simulink model "Manual_Simu_2022a"  (R2022a)
settings: Solver=VariableStepAuto  StartTime=0.0  StopTime=3  RelTol=1e-3
values from neighbouring files (symbols this model uses):
  c = 0.9    [Mechatronics_System.m]
  g = 9.81    [Mechatronics_System.m]
  I_p = (1/3)*m_p*l^2    (= 2.35225)    [Mechatronics_System.m]
  l = 0.97    [Mechatronics_System.m]
  m_p = 7.5    [Mechatronics_System.m]
  m_w = 30.5    [Mechatronics_System.m]
libraries: simulink_extras x2, simulink x1
settings Model: Creator=sango  LastModifiedBy=sango
settings DebuggingCC: ArtificialAlgebraicLoopMsg=none
settings ModelReferenceCC: EnableRefExpFcnMdlSchedulingChecks=off
settings RTWCC: Description=Generic Real-Time Target

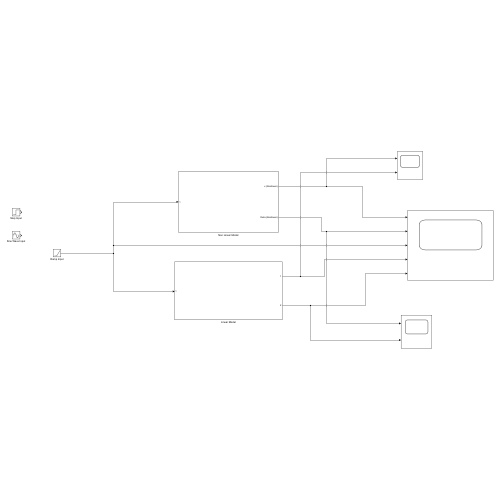
[thumbnail: Simulink's stored preview of the top-level diagram]
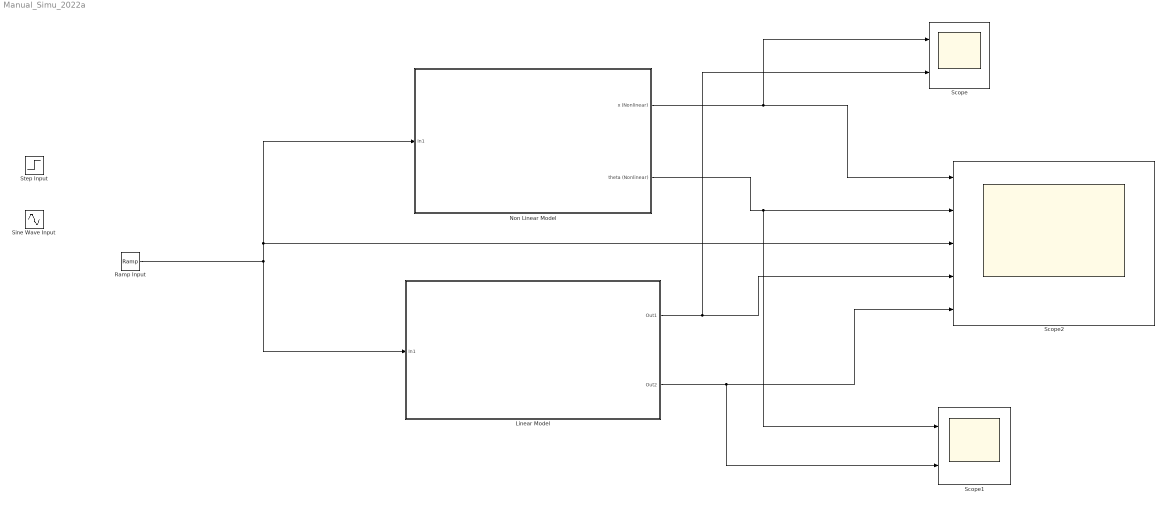
== system Manual_Simu_2022a ==
  Linear Model : Subsystem
  Non Linear Model : Subsystem
  Ramp Input : simulink/Sources/Ramp  slope=2  start=0  InitialOutput=0
  Scope : Scope  NumInputPorts=2
  Scope1 : Scope  NumInputPorts=2
  Scope2 : Scope  NumInputPorts=5
  Sine Wave Input : Sin  SampleTime=0
  Step Input : Step  SampleTime=0
  wires:
  Non Linear Model/1(x (Nonlinear)) -> Scope/1, Scope2/1
  Non Linear Model/2(theta (Nonlinear)) -> Scope1/1, Scope2/2
  Ramp Input/1 -> Linear Model/1(In1), Scope2/3, Non Linear Model/1(In1)
  Linear Model/1(Out1) -> Scope/2, Scope2/4
  Linear Model/2(Out2) -> Scope1/2, Scope2/5

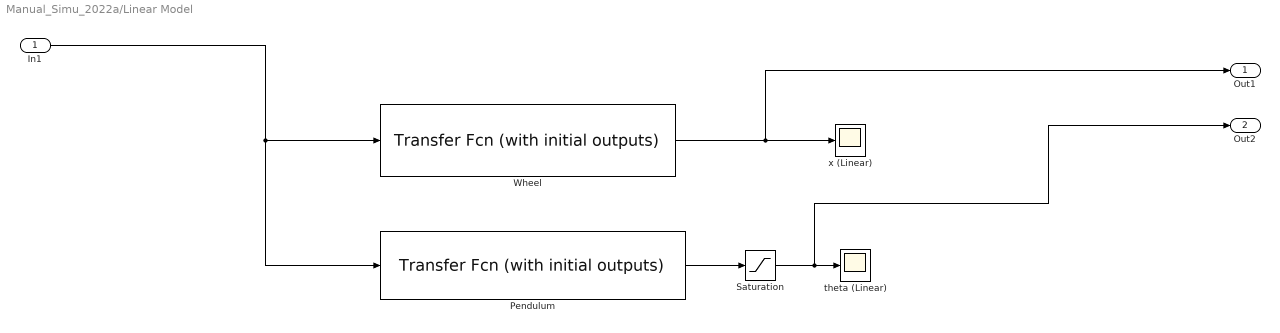
== system Manual_Simu_2022a/Linear Model ==
  In1 : Inport
  Pendulum : simulink_extras/Additional Linear/Transfer Fcn (with initial outputs)  N=[6.751e05 0]  D="[2.827e07 7.858e05 -2.516e08  -5.96e06]"  Y0=pi/2  U0=0
  Saturation : Saturate  UpperLimit=pi  LowerLimit=0
  Wheel : simulink_extras/Additional Linear/Transfer Fcn (with initial outputs)  N=[8.731e05 0 -6.622e06]  D=[2.827e07 7.858e05 -2.516e08 -5.96e06 0]  Y0=0  U0=0
  theta (Linear) : Scope
  x (Linear) : Scope
  Out1 : Outport
  Out2 : Outport  Port=2
  wires:
  Pendulum/1 -> Saturation/1
  Saturation/1 -> Out2/1, theta (Linear)/1
  Wheel/1 -> Out1/1, x (Linear)/1
  In1/1 -> Pendulum/1, Wheel/1

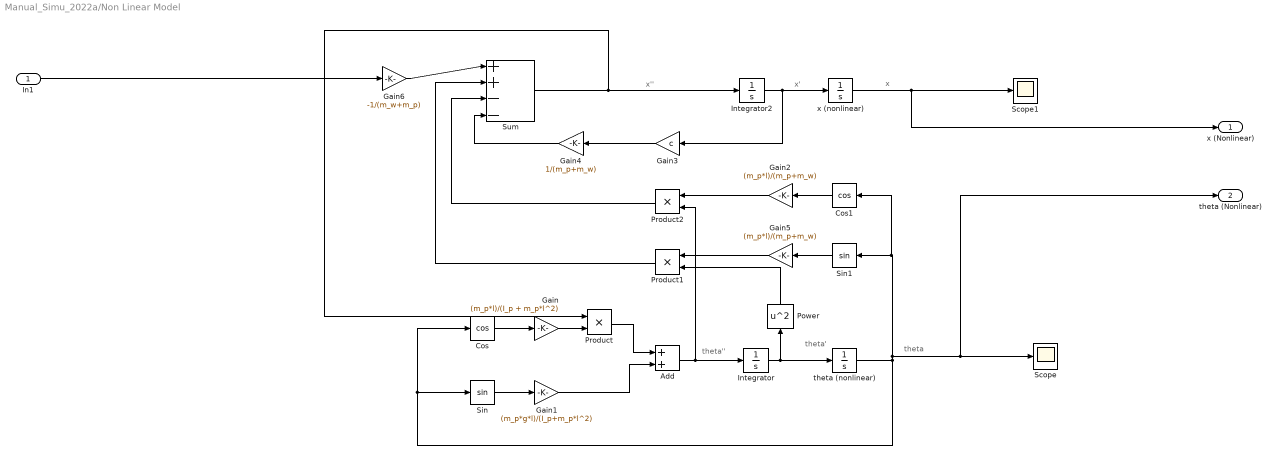
== system Manual_Simu_2022a/Non Linear Model ==
  note: x''
  note: x'
  note: x
  note: theta
  note: theta'
  note: theta''
  In1 : Inport
  Add : Sum
  Cos : Trigonometry  Operator=cos
  Cos1 : Trigonometry  Operator=cos
  Gain : Gain  Gain=(m_p*l)/(I_p + m_p*l^2)
  Gain1 : Gain  Gain=(m_p*g*l)/(I_p+m_p*l^2)
  Gain2 : Gain  Gain=(m_p*l)/(m_p+m_w)
  Gain3 : Gain  Gain=c
  Gain4 : Gain  Gain=1/(m_p+m_w)
  Gain5 : Gain  Gain=(m_p*l)/(m_p+m_w)
  Gain6 : Gain  Gain=-1/(m_w+m_p)
  Integrator : Integrator
  Integrator2 : Integrator
  Power : Math  Operator=square
  Product : Product
  Product1 : Product
  Product2 : Product
  Scope : Scope
  Scope1 : Scope
  Sin : Trigonometry
  Sin1 : Trigonometry
  Sum : Sum  Inputs=|++--
  theta (nonlinear) : Integrator  InitialCondition=pi/2  LimitOutput=on  UpperSaturationLimit=pi  LowerSaturationLimit=0  ContinuousStateAttributes='theta'
  x (nonlinear) : Integrator
  x (Nonlinear) : Outport
  theta (Nonlinear) : Outport  Port=2
  wires:
  Gain/1 -> Product/2
  theta (nonlinear)/1 -> theta (Nonlinear)/1, Scope/1, Cos1/1, Sin1/1, Sin/1, Cos/1
  Power/1 -> Product1/2
  Sin/1 -> Gain1/1
  Gain1/1 -> Add/2
  Add/1 -> Product2/2, Integrator/1
  Cos/1 -> Gain/1
  Integrator2/1 -> Gain3/1, x (nonlinear)/1
  Integrator/1 -> theta (nonlinear)/1, Power/1
  Sum/1 -> Integrator2/1, Product/1
  In1/1 -> Gain6/1
  x (nonlinear)/1 -> x (Nonlinear)/1, Scope1/1
  Product/1 -> Add/1
  Product1/1 -> Sum/2
  Product2/1 -> Sum/3
  Sin1/1 -> Gain5/1
  Gain2/1 -> Product2/1
  Gain3/1 -> Gain4/1
  Cos1/1 -> Gain2/1
  Gain4/1 -> Sum/4
  Gain5/1 -> Product1/1
  Gain6/1 -> Sum/1
